simulink model "part13"  (R2017b)
settings: Solver=VariableStepAuto  StartTime=0.0  StopTime=10  RelTol=1e-3
settings Model: Creator=admin  LastModifiedBy=admin

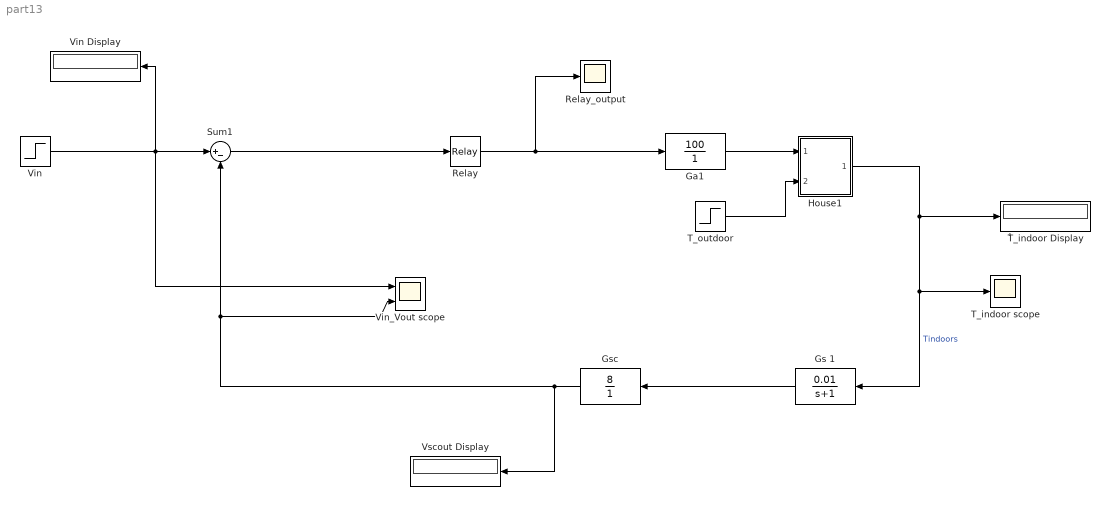
== system part13 ==
  Ga1 : TransferFcn  Numerator=[100]  Denominator=[1 ]
  Gs 1 : TransferFcn  Numerator=[0.01]  Denominator=[1 1]
  Gsc : TransferFcn  Numerator=[8]  Denominator=[1 ]
  House1 : Subsystem
      mask Display: image(fullfile(matlabroot,'toolbox','simulink','simdemos','simgeneral','images','HouseHeatHousePix.svg'))
  Relay : Relay  OnOutputValue=10
  "Relay_output " : Scope
  Sum1 : Sum  Inputs=|+-
  "T_indoor scope " : Scope
  "T_outdoor " : Step  Time=0  After=15  SampleTime=0
  "Vin " : Step  Time=0  After=2.06  SampleTime=0
  "Vin Display " : Display
  "Vin_Vout scope " : Scope  NumInputPorts=2
  "Vscout Display " : Display
  ْT_indoor Display : Display
  wires:
  "T_outdoor "/1 -> House1/2(Outdoor Temp Tout)
  Gsc/1 -> Sum1/2, "Vin_Vout scope "/2, "Vscout Display "/1
  Ga1/1 -> House1/1(Heater QDot In)
  House1/1(Room Temp Troom) -> ْT_indoor Display/1, "T_indoor scope "/1, Gs 1/1  "Tindoors"
  Gs 1/1 -> Gsc/1
  Relay/1 -> Ga1/1, "Relay_output "/1
  Sum1/1 -> Relay/1
  "Vin "/1 -> "Vin Display "/1, Sum1/1, "Vin_Vout scope "/1

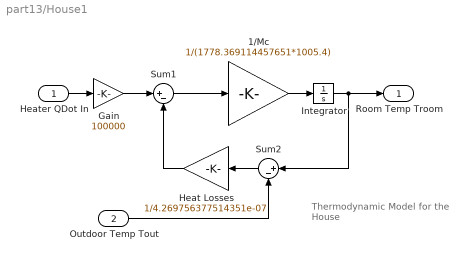
== system part13/House1 ==
  note: Thermodynamic Model
      | for the House
  Heater QDot In : Inport
  Outdoor Temp Tout : Inport  Port=2
  1/Mc : Gain  Gain=1/(1778.369114457651*1005.4)  SaturateOnIntegerOverflow=on  OutDataTypeStr=Inherit: Same as input  ParamDataTypeStr=Inherit: Same as input
  Gain : Gain  Gain=100000
  Heat Losses : Gain  Gain=1/4.269756377514351e-07  SaturateOnIntegerOverflow=on  OutDataTypeStr=Inherit: Same as input  ParamDataTypeStr=Inherit: Same as input
  Integrator : Integrator  InitialCondition=20
  Sum1 : Sum  Inputs=|+-  SaturateOnIntegerOverflow=on  InputSameDT=on  OutDataTypeStr=Inherit: Same as first input
  Sum2 : Sum  Inputs=|+-  SaturateOnIntegerOverflow=on  InputSameDT=on  OutDataTypeStr=Inherit: Same as first input
  Room Temp Troom : Outport  InitialOutput=0
  wires:
  Outdoor Temp Tout/1 -> Sum2/2
  Heater QDot In/1 -> Gain/1
  Sum1/1 -> 1/Mc/1
  Sum2/1 -> Heat Losses/1
  Heat Losses/1 -> Sum1/2
  1/Mc/1 -> Integrator/1
  Integrator/1 -> Sum2/1, Room Temp Troom/1
  Gain/1 -> Sum1/1
